simulink model "QBot2_Integration_Sensors_2017"  (Simulink 8.9)
settings: Solver=FixedStepDiscrete  StartTime=0.0  StopTime=inf  FixedStep=0.01  RelTol=1e-3  EnableMultiTasking=on
undefined symbols (not defined in the file): HIL
libraries: quarc_library x5
settings Model: Creator=drmadill  LastModifiedBy=amolki  SimulationMode=external  ExtModeTrigDuration=1
settings SolverCC: PositivePriorityOrder=on
settings OptimizationCC: ExpressionDepthLimit=2147483647  LifeSpan=auto
settings DebuggingCC: SolverPrmCheckMsg=warning
settings RTWCC: SystemTargetFile=quarc_linux_pi_3.tlc  TemplateMakefile=quarc_linux_pi_3_tmf  Description=QUARC Linux Raspberry Pi 3 Target
settings STFCustomTargetCC: TargetLibSuffix=.a  TargetPreCompLibLocation=C:\PROGRA~3\QUARC\lib\2018a\LINUX_~4\release  ConcurrentExecutionCompliant=on  SystemTargetFile=quarc_linux_pi_3.tlc
settings GRTTargetCC: TargetLibSuffix=.a  TargetPreCompLibLocation=C:\PROGRA~3\QUARC\lib\2018a\LINUX_~4\release  ParMdlRefBuildCompliant=off  CompOptLevelCompliant=off  GeneratePreprocessorConditionals=Use local settings  MatFileLogging=off  CPPClassGenCompliant=off  UseToolchainInfoCompliant=off  ExtMode=on  ExtModeMexFile=quarc_comm  ExtModeMexArgs='-w -d /tmp -uri %u'
settings ConfigComp: CovSFcnEnable=off

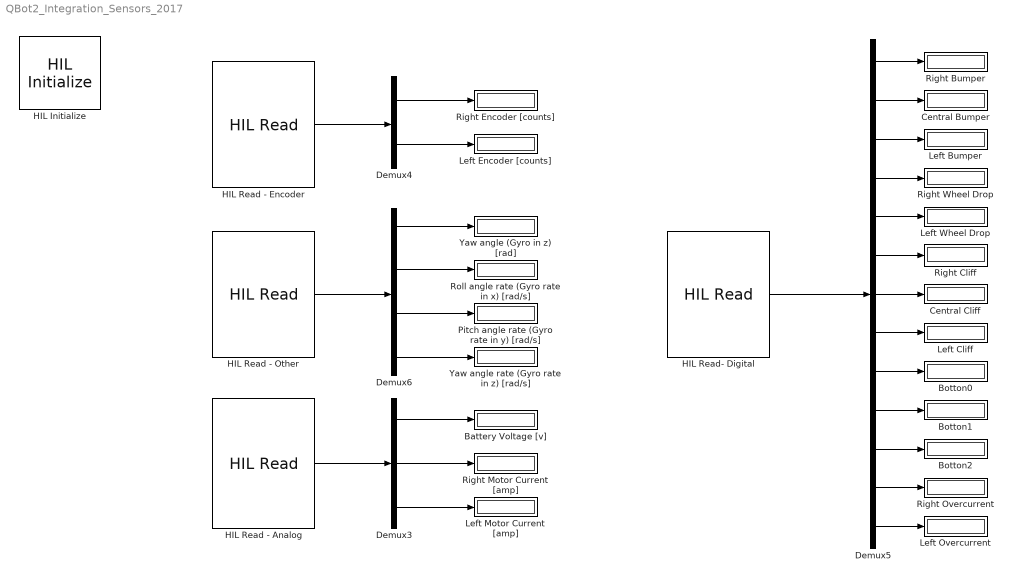
== system QBot2_Integration_Sensors_2017 ==
  Battery Voltage [v] : Display
      settings: Decimation=20
  Botton0 : Display
      settings: Decimation=20
  Botton1 : Display
      settings: Decimation=20
  Botton2 : Display
      settings: Decimation=20
  Central Bumper : Display
      settings: Decimation=20
  Central Cliff : Display
      settings: Decimation=20
  Demux3 : Demux  Outputs=3
  Demux4 : Demux  Outputs=2
  Demux5 : Demux  Outputs=13
  Demux6 : Demux
  HIL Initialize : quarc_library/Data Acquisition/Generic/Configuration/HIL Initialize  Priority=-99  object_name=HIL-1  board_type=qbot2e  board_number=0  board_options=pwm0_en=1;pwm0_pin=12;pwm1_en=1;pwm1_pin=13;  exclusive=off  active=off  hardware_clocks=[]  clock_modes=[]  initial_clock_frequencies=[]  set_clock_params_at_start=off  set_clock_params_at_switch_in=off  set_clock_frequencies_at_start=off  set_clock_frequencies_at_switch_in=off  analog_input_channels=[0:5]  analog_input_configurations=[]  analog_input_maximums=[16.5 3.3 3.3 3.3 3.3 3.3]  analog_input_minimums=[0 0 0 0 0 0]  set_analog_input_params_at_start=off  set_analog_input_params_at_switch_in=off  analog_output_channels=[]  analog_output_maximums=[]  analog_output_minimums=[]  initial_analog_outputs=[]  final_analog_outputs=[]  watchdog_analog_outputs=[]  set_analog_output_params_at_start=off  set_analog_output_params_at_switch_in=off  set_analog_outputs_at_start=off  set_analog_outputs_at_switch_in=off  set_analog_outputs_at_terminate=off  set_analog_outputs_at_switch_out=off  set_analog_outputs_on_watchdog=off  digital_input_channels=[28:58]  digital_output_channels=[28:31]  digital_output_configuration=[]  initial_digital_outputs=[0]  final_digital_outputs=[0]  watchdog_digital_outputs=[]  set_digital_output_params_at_start=off  set_digital_output_params_at_switch_in=off  set_digital_outputs_at_start=on  set_digital_outputs_at_switch_in=off  set_digital_outputs_at_terminate=on  set_digital_outputs_at_switch_out=off  set_digital_outputs_on_watchdog=off  encoder_channels=[0:1]  quadrature=[4]  encoder_filter_frequency=[]  initial_encoder_counts=[0]  set_encoder_params_at_start=on  set_encoder_params_at_switch_in=off  set_encoder_counts_at_start=on  set_encoder_counts_at_switch_in=off  pwm_channels=[0:1]  pwm_modes=0  pwm_frequency=100e6 / 4095  pwm_configuration=[0]  pwm_alignment=[0]  pwm_polarity=[1]  pwm_leading_deadband=[]  pwm_trailing_deadband=[]  initial_pwm_outputs=[0]  final_pwm_outputs=[0]  watchdog_pwm_outputs=[]  set_pwm_params_at_start=on  set_pwm_params_at_switch_in=off  set_pwm_outputs_at_start=on  set_pwm_outputs_at_switch_in=off  set_pwm_outputs_at_terminate=on  set_pwm_outputs_at_switch_out=off  set_pwm_outputs_on_watchdog=off  other_output_channels=[2000:2001 14000 16000]  initial_other_outputs=[0 0 0 7]  final_other_outputs=[0 0 0 7]  watchdog_other_outputs=[]  set_other_outputs_at_start=on  set_other_outputs_at_switch_in=off  set_other_outputs_at_terminate=on  set_other_outputs_at_switch_out=off  set_other_outputs_on_watchdog=off
  HIL Read - Analog : quarc_library/Data Acquisition/Generic/Immediate I//O/HIL Read  object_name=HIL-1  analog_channels=[0 4:5]  encoder_channels=[]  digital_channels=[]  other_channels=[]  sample_time=qc_get_step_size  active=on  vector_output=on  data_type_mode=Inherit via back propagation  encoder_data_type=double  digital_data_type=boolean
  HIL Read - Encoder : quarc_library/Data Acquisition/Generic/Immediate I//O/HIL Read  object_name=HIL-1  analog_channels=[]  encoder_channels=[0:1]  digital_channels=[]  other_channels=[]  sample_time=qc_get_step_size  active=on  vector_output=on  data_type_mode=Inherit via back propagation  encoder_data_type=double  digital_data_type=boolean
  HIL Read - Other : quarc_library/Data Acquisition/Generic/Immediate I//O/HIL Read  object_name=HIL-1  analog_channels=[]  encoder_channels=[]  digital_channels=[]  other_channels=[1002 3000:3002]  sample_time=qc_get_step_size  active=on  vector_output=on  data_type_mode=Inherit via back propagation  encoder_data_type=double  digital_data_type=boolean
  HIL Read- Digital : quarc_library/Data Acquisition/Generic/Immediate I//O/HIL Read  object_name=HIL-1  analog_channels=[]  encoder_channels=[]  digital_channels=[28:40]  other_channels=[]  sample_time=qc_get_step_size  active=on  vector_output=on  data_type_mode=Inherit via back propagation  encoder_data_type=double  digital_data_type=boolean
  Left Bumper : Display
      settings: Decimation=20
  Left Cliff : Display
      settings: Decimation=20
  Left Encoder [counts] : Display
      settings: Decimation=20
  Left Motor Current [amp] : Display
      settings: Decimation=20
  Left Overcurrent : Display
      settings: Decimation=20
  Left Wheel Drop : Display
      settings: Decimation=20
  Pitch angle rate (Gyro rate in y) [rad/s] : Display
      settings: Decimation=20
  Right Bumper : Display
      settings: Decimation=20
  Right Cliff : Display
      settings: Decimation=20
  Right Encoder [counts] : Display
      settings: Decimation=20
  Right Motor Current [amp] : Display
      settings: Decimation=20
  Right Overcurrent : Display
      settings: Decimation=20
  Right Wheel Drop : Display
      settings: Decimation=20
  Roll angle rate (Gyro rate in x) [rad/s] : Display
      settings: Decimation=20
  Yaw angle (Gyro in z) [rad] : Display
      settings: Decimation=20
  Yaw angle rate (Gyro rate in z) [rad/s] : Display
      settings: Decimation=20
  wires:
  HIL Read - Analog/1 -> Demux3/1
  Demux3/1 -> Battery Voltage [v]/1
  Demux3/2 -> Right Motor Current [amp]/1
  Demux3/3 -> Left Motor Current [amp]/1
  Demux4/1 -> Right Encoder [counts]/1
  Demux4/2 -> Left Encoder [counts]/1
  HIL Read - Encoder/1 -> Demux4/1
  HIL Read- Digital/1 -> Demux5/1
  Demux5/2 -> Central Bumper/1
  Demux5/3 -> Left Bumper/1
  Demux5/4 -> Right Wheel Drop/1
  Demux5/5 -> Left Wheel Drop/1
  Demux5/6 -> Right Cliff/1
  Demux5/7 -> Central Cliff/1
  Demux5/8 -> Left Cliff/1
  Demux5/9 -> Botton0/1
  Demux5/10 -> Botton1/1
  Demux5/11 -> Botton2/1
  Demux5/12 -> Right Overcurrent/1
  Demux5/13 -> Left Overcurrent/1
  HIL Read - Other/1 -> Demux6/1
  Demux6/1 -> Yaw angle (Gyro in z) [rad]/1
  Demux6/2 -> Roll angle rate (Gyro rate in x) [rad/s]/1
  Demux5/1 -> Right Bumper/1
  Demux6/3 -> Pitch angle rate (Gyro rate in y) [rad/s]/1
  Demux6/4 -> Yaw angle rate (Gyro rate in z) [rad/s]/1
